simulink model "TUD_impedanceControl"  (Simulink 7.9)
settings: Solver=FixedStepDiscrete  StartTime=0.0  StopTime=inf  FixedStep=Ts  RelTol=1e-3
InitFcn:
  | config;
  | perturbation;
values from neighbouring files (symbols this model uses):
  tau_p = [torso_pitch; torso_roll; torso_yaw; left_shoulder_pitch; left_shoulder_roll; left_shoulder_yaw; left_elbow; left_wrist_prosup;      right_shoulder_pitch; right_shoulder_roll; right_shoulder_yaw; right_elbow; right_wrist_prosup; left_hip_pitch; left_hip_roll;      left_hip_yaw; left_knee; left_ankle_pitch; left_ankle_roll; right_hip_pitch;  right_hip_roll; right_hip_yaw; right_knee; right_ankle_pi ...(+22 chars)    [initialisation.m]    (also in perturbation.m)
  Tm_t = 50    [initialisation.m]    (also in perturbation.m)
  Ts = 0.1    [initialisation.m]    (also in perturbation.m)
libraries: WBCLibrary x7
settings Model: Creator=labar  LastModifiedBy=labar

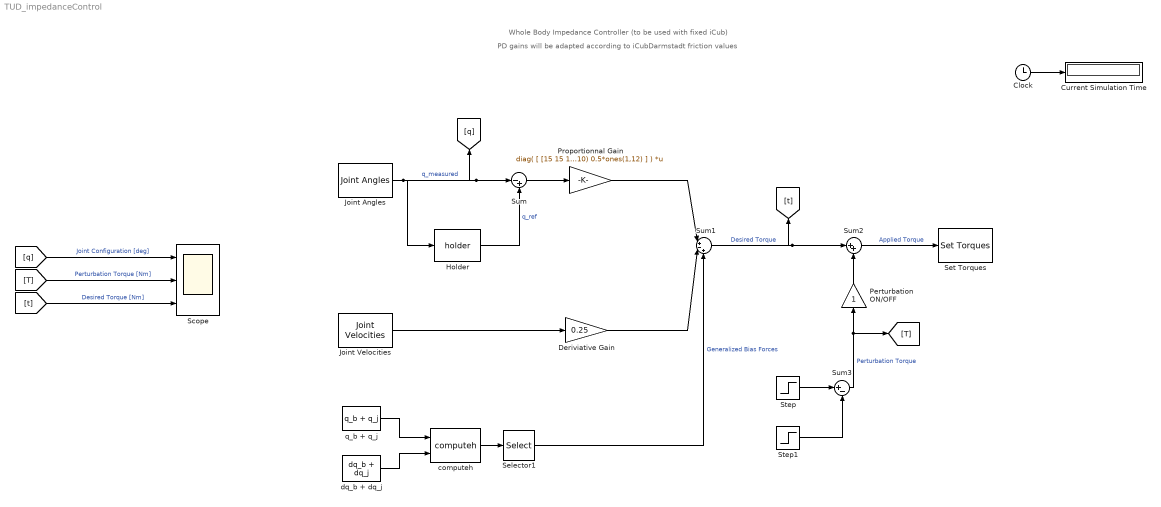
== system TUD_impedanceControl ==
  note: Whole Body Impedance Controller (to be used with fixed iCub)
  note: PD gains will be adapted according to iCubDarmstadt friction values
  Clock : Clock
  Current Simulation Time : Display
  Deriviative Gain : Gain  Gain=0.25
  Holder : WBCLibrary/Utilities/holder 
  Joint Angles : WBCLibrary/wholeBodyStates/Joint Angles  robotName=robotName  localName=localName
  Joint Velocities : WBCLibrary/wholeBodyStates/Joint Velocities  robotName=robotName  localName=localName
  Perturbation ON/OFF : Gain
  Proportionnal Gain : Gain  Gain=diag( [ [15 15 15] 2*ones(1,10) 0.5*ones(1,12) ] )  Multiplication=Matrix(K*u)
  Scope : Scope  NumInputPorts=3
      settings: ShowLegends=on  YMin=-5~-5~-5  YMax=5~5~5
  Selector1 : Selector  InputPortWidth=31  IndexOptions=Index vector (dialog)  Indices=[7:31]  OutputSizes=1
  Set Torques : WBCLibrary/wholeBodyActuators/Set Torques  val=6  robotName=robotName  localName=localName
  Step : Step  Time=10  Before=zeros(1,25)  After=tau_p  SampleTime=0
  Step1 : Step  Time=10+Tm_t  Before=zeros(1,25)  After=tau_p  SampleTime=0
  Sum : Sum  Inputs=|-+
  Sum1 : Sum  Inputs=|+-+
  Sum2 : Sum  Inputs=|++
  Sum3 : Sum  Inputs=|+-
  computeh : WBCLibrary/wholeBodyModel/Dynamics/computeh  val=7  robotname=robotName  localname=localName
  dq_b + dq_j : WBCLibrary/wholeBodyStates/dq_b + dq_j  robotName=robotName  localName=localName  Ts=Ts
  q_b + q_j : WBCLibrary/wholeBodyStates/q_b + q_j  robotName=robotName  localName=localName  Ts=Ts
  wires:
  Joint Angles/1 -> Holder/1, Sum/1, [q]  "q_measured"
  Holder/1 -> Sum/2  "q_ref"
  Joint Velocities/1 -> Deriviative Gain/1
  Sum/1 -> Proportionnal Gain/1
  Proportionnal Gain/1 -> Sum1/1
  Deriviative Gain/1 -> Sum1/2
  q_b + q_j/1 -> computeh/1
  dq_b + dq_j/1 -> computeh/2
  computeh/1 -> Selector1/1
  Sum1/1 -> Sum2/1, [t]  "Desired Torque"
  Step1/1 -> Sum3/2
  Step/1 -> Sum3/1
  Sum3/1 -> Perturbation ON/OFF/1, [T]  "Perturbation Torque"
  Sum2/1 -> Set Torques/1  "Applied Torque"
  Selector1/1 -> Sum1/3  "Generalized Bias Forces"
  Perturbation ON/OFF/1 -> Sum2/2
  [T] -> Scope/2  "Perturbation Torque [Nm]"
  [q] -> Scope/1  "Joint Configuration [deg]"
  [t] -> Scope/3  "Desired Torque [Nm]"
  Clock/1 -> Current Simulation Time/1
